simulink model "Traj2"  (R2025b)
settings: Solver=FixedStepAuto  StartTime=0.0  StopTime=inf  RelTol=1e-3
values from neighbouring files (symbols this model uses):
  K = [2.2361, 0, 0; 0, 2.8868, 2.5456]    [lq.m]
  vd_ref = v_refs    [lq.m]    (also in run_planner.m = zeros(N, 1))
  wd_ref = w_refs    [lq.m]    (also in run_planner.m = zeros(N, 1))
undefined symbols (not defined in the file or in its folder): L, P, theta0, theta_ref_unwrapped, Ts_ref, x0, y0
libraries: simulink x4, slpidlib x2
settings Model: Creator=mwali  LastModifiedBy=hassa
settings OptimizationCC: FunctionInliningControlUserFunctions=Never  FunctionInliningControlMWFunctions=Readability  FunctionInliningControlMWUserFunctions=Never  OptimizeBlockIOStorage=off  OptimizeDataStoreBuffers=off  BusAssignmentInplaceUpdate=off
settings DebuggingCC: SFUnexpectedBacktrackingDiag=warning  SFNoUnconditionalDefaultTransitionDiag=warning
settings RTWCC: GenerateReport=on  BuildConfiguration=Debug  LaunchReport=on
settings CodeAppCC: ForceParamTrailComments=on  MATLABSourceComments=on  EnableCustomComments=on
settings GRTTargetCC: MultiInstanceErrorCode=Warning  CombineSignalStateStructs=on  SupportVariableSizeSignals=on

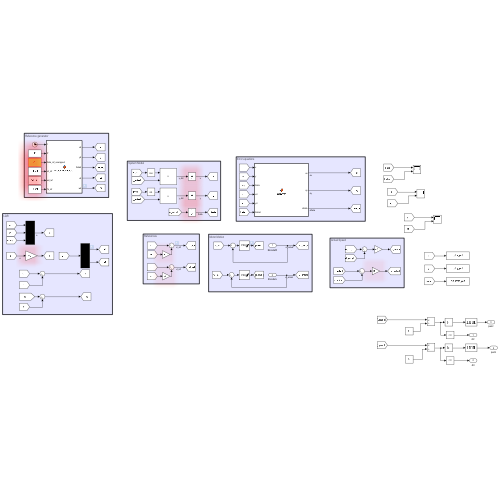
[thumbnail: Simulink's stored preview of the top-level diagram]
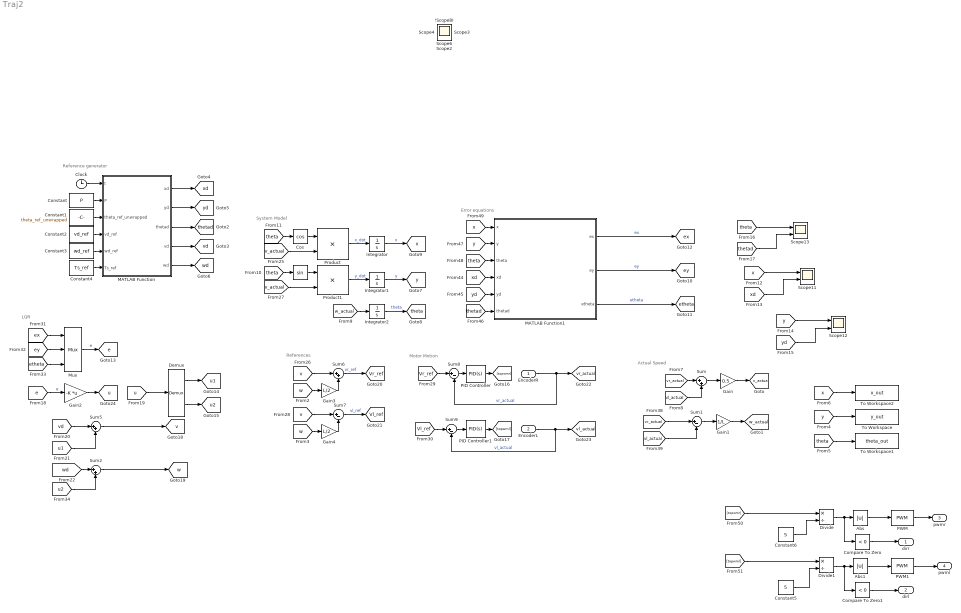
== system Traj2 ==
  note: Error equations
  note: Actual Speed
  note: Motor Motion
  note: References
  note: LQR
  note: System Model
  note: Reference generator
  EncoderR : Inport
  EncoderL : Inport  Port=2
  " " : Trigonometry
  Abs : Abs  SaturateOnIntegerOverflow=off
  Abs1 : Abs  SaturateOnIntegerOverflow=off
  Clock : Clock
  Compare To Zero : simulink/Logic and Bit Operations/Compare To Zero  relop=<  OutDataTypeStr=boolean
  Compare To Zero1 : simulink/Logic and Bit Operations/Compare To Zero  relop=<  OutDataTypeStr=boolean
  Constant : Constant  Value=P
  Constant1 : Constant  Value=theta_ref_unwrapped
  Constant2 : Constant  Value=vd_ref
  Constant3 : Constant  Value=wd_ref
  Constant4 : Constant  Value=Ts_ref
  Constant5 : Constant  Value=5
  Constant6 : Constant  Value=5
  Cos : Trigonometry  Operator=cos
  Demux : Demux  Outputs=2
  Divide : Product  Inputs=*/
  Divide1 : Product  Inputs=*/
  Gain : Gain  Gain=0.5
  Gain1 : Gain  Gain=1/L
  Gain2 : Gain  Gain=-K  Multiplication=Matrix(K*u)
  Gain3 : Gain  Gain=L/2
  Gain4 : Gain  Gain=L/2
  Integrator : Integrator  InitialCondition=x0
  Integrator1 : Integrator  InitialCondition=y0
  Integrator2 : Integrator  InitialCondition=theta0
  MATLAB Function : MATLAB Function  TreatAsAtomicUnit=on
  MATLAB Function1 : MATLAB Function  TreatAsAtomicUnit=on
  Mux : Mux  Inputs=3
  PID Controller : slpidlib/PID Controller  Controller=PID  Form=Parallel  TimeDomain=Continuous-time  UseExternalTs=off  SampleTime=-1  IntegratorMethod=Forward Euler  FilterMethod=Forward Euler  ControllerParametersSource=internal  P=5  I=20  UseKiTs=off  D=0  UseExternalDerivativeSource=off  N=100  UseFilter=on  TunerSelectOption=Transfer Function Based (PID Tuner App)  InitialConditionSource=internal  InitialConditionForIntegrator=0  InitialConditionForFilter=0  DifferentiatorICPrevScaledInput=0  ExternalReset=none  TrackingMode=off  Kt=1  LimitOutput=on  SatLimitsSource=internal  UpperSaturationLimit=5  LowerSaturationLimit=-5  LinearizeAsGain=on  AntiWindupMode=clamping  Kb=1  LimitIntegrator=off  UpperIntegratorSaturationLimit=inf  LowerIntegratorSaturationLimit=-inf  POutMin=[]  POutMax=[]  IOutMin=[]  IOutMax=[]  DOutMin=[]  DOutMax=[]  NOutMin=[]  NOutMax=[]  SumOutMin=[]  SumOutMax=[]  SaturationOutMin=[]  SaturationOutMax=[]  PParamMin=[]  PParamMax=[]  IParamMin=[]  IParamMax=[]  DParamMin=[]  DParamMax=[]  NParamMin=[]  NParamMax=[]  KbParamMin=[]  KbParamMax=[]  KtParamMin=[]  KtParamMax=[]  KbOutMin=[]  KbOutMax=[]  KtOutMin=[]  KtOutMax=[]  IntegratorOutMin=[]  IntegratorOutMax=[]  FilterOutMin=[]  FilterOutMax=[]  SumI1OutMin=[]  SumI1OutMax=[]  SumI2OutMin=[]  SumI2OutMax=[]  SumI3OutMin=[]  SumI3OutMax=[]  SumI4OutMin=[]  SumI4OutMax=[]  SumDOutMin=[]  SumDOutMax=[]  DifferentiatorOutMin=[]  DifferentiatorOutMax=[]  FilterDiffOutCoefMin=[]  FilterDiffOutCoefMax=[]  ReciprocalOutMin=[]  ReciprocalOutMax=[]  SumDenOutMin=[]  SumDenOutMax=[]  SumNumOutMin=[]  SumNumOutMax=[]  DivideOutMin=[]  DivideOutMax=[]  UdiffTsProdOutMin=[]  UdiffTsProdOutMax=[]  NTsProdOutMin=[]  NTsProdOutMax=[]  UintegralTsProdOutMin=[]  UintegralTsProdOutMax=[]  UngainTsProdOutMin=[]  UngainTsProdOutMax=[]  ClampingZeroOutDataTypeStr=Inherit: Inherit via back propagation  ClampingZeroOutMin=[]  ClampingZeroOutMax=[]  FilterDenConstantOutDataTypeStr=Inherit: Inherit via back propagation  FilterDenConstantOutMin=[]  FilterDenConstantOutMax=[]  PCopyOutDataTypeStr=Inherit: Inherit via back propagation  PCopyOutMin=[]  PCopyOutMax=[]  NCopyOutDataTypeStr=Inherit: Inherit via back propagation  NCopyOutMin=[]  NCopyOutMax=[]  IntegratorContinuousStateAttributes=''  IntegratorStateMustResolveToSignalObject=off  IntegratorRTWStateStorageClass=Auto  FilterContinuousStateAttributes=''  FilterStateMustResolveToSignalObject=off  FilterRTWStateStorageClass=Auto  ParallelPVariant=InternalParameters  IdealPVariant=Disabled  IVariant=InternalParameters  DVariant=InternalParameters  IntegratorVariant=Continuous  SatVariant=Enabled  AWVariant=ContClampingParallel  PCopyVariant=Disabled  TRVariant=Disabled  FdbkBlocksVariant=Forward  IdealPFdbkVariant=Disabled  SatFdbkVariant=Disabled  DerivativeFilterVariant=ContFilter  NVariant=InternalParameters  NCopyVariant=Disabled  FilterICVariant=InternalICsFilter  IntegratorICVariant=InternalICs  ExternalResetVariant=Disabled  TRSumVariant=Passthrough  SumFdbkVariant=Disabled  SumVariant=Sum_PID  TsampFilterVariant=InternalTs  TsampNgainVariant=Passthrough  TsampIntegralVariant=Disabled_SignalSpec  ExternalSaturationOutDataTypeStr=Inherit: Same as second input  DerivativeSourceVariant=ErrorSignal  PreIntVariant=InternalPreInt
  PID Controller1 : slpidlib/PID Controller  Controller=PID  Form=Parallel  TimeDomain=Continuous-time  UseExternalTs=off  SampleTime=-1  IntegratorMethod=Forward Euler  FilterMethod=Forward Euler  ControllerParametersSource=internal  P=5  I=20  UseKiTs=off  D=0  UseExternalDerivativeSource=off  N=100  UseFilter=on  TunerSelectOption=Transfer Function Based (PID Tuner App)  InitialConditionSource=internal  InitialConditionForIntegrator=0  InitialConditionForFilter=0  DifferentiatorICPrevScaledInput=0  ExternalReset=none  TrackingMode=off  Kt=1  LimitOutput=on  SatLimitsSource=internal  UpperSaturationLimit=5  LowerSaturationLimit=-5  LinearizeAsGain=on  AntiWindupMode=clamping  Kb=1  LimitIntegrator=off  UpperIntegratorSaturationLimit=inf  LowerIntegratorSaturationLimit=-inf  POutMin=[]  POutMax=[]  IOutMin=[]  IOutMax=[]  DOutMin=[]  DOutMax=[]  NOutMin=[]  NOutMax=[]  SumOutMin=[]  SumOutMax=[]  SaturationOutMin=[]  SaturationOutMax=[]  PParamMin=[]  PParamMax=[]  IParamMin=[]  IParamMax=[]  DParamMin=[]  DParamMax=[]  NParamMin=[]  NParamMax=[]  KbParamMin=[]  KbParamMax=[]  KtParamMin=[]  KtParamMax=[]  KbOutMin=[]  KbOutMax=[]  KtOutMin=[]  KtOutMax=[]  IntegratorOutMin=[]  IntegratorOutMax=[]  FilterOutMin=[]  FilterOutMax=[]  SumI1OutMin=[]  SumI1OutMax=[]  SumI2OutMin=[]  SumI2OutMax=[]  SumI3OutMin=[]  SumI3OutMax=[]  SumI4OutMin=[]  SumI4OutMax=[]  SumDOutMin=[]  SumDOutMax=[]  DifferentiatorOutMin=[]  DifferentiatorOutMax=[]  FilterDiffOutCoefMin=[]  FilterDiffOutCoefMax=[]  ReciprocalOutMin=[]  ReciprocalOutMax=[]  SumDenOutMin=[]  SumDenOutMax=[]  SumNumOutMin=[]  SumNumOutMax=[]  DivideOutMin=[]  DivideOutMax=[]  UdiffTsProdOutMin=[]  UdiffTsProdOutMax=[]  NTsProdOutMin=[]  NTsProdOutMax=[]  UintegralTsProdOutMin=[]  UintegralTsProdOutMax=[]  UngainTsProdOutMin=[]  UngainTsProdOutMax=[]  ClampingZeroOutDataTypeStr=Inherit: Inherit via back propagation  ClampingZeroOutMin=[]  ClampingZeroOutMax=[]  FilterDenConstantOutDataTypeStr=Inherit: Inherit via back propagation  FilterDenConstantOutMin=[]  FilterDenConstantOutMax=[]  PCopyOutDataTypeStr=Inherit: Inherit via back propagation  PCopyOutMin=[]  PCopyOutMax=[]  NCopyOutDataTypeStr=Inherit: Inherit via back propagation  NCopyOutMin=[]  NCopyOutMax=[]  IntegratorContinuousStateAttributes=''  IntegratorStateMustResolveToSignalObject=off  IntegratorRTWStateStorageClass=Auto  FilterContinuousStateAttributes=''  FilterStateMustResolveToSignalObject=off  FilterRTWStateStorageClass=Auto  ParallelPVariant=InternalParameters  IdealPVariant=Disabled  IVariant=InternalParameters  DVariant=InternalParameters  IntegratorVariant=Continuous  SatVariant=Enabled  AWVariant=ContClampingParallel  PCopyVariant=Disabled  TRVariant=Disabled  FdbkBlocksVariant=Forward  IdealPFdbkVariant=Disabled  SatFdbkVariant=Disabled  DerivativeFilterVariant=ContFilter  NVariant=InternalParameters  NCopyVariant=Disabled  FilterICVariant=InternalICsFilter  IntegratorICVariant=InternalICs  ExternalResetVariant=Disabled  TRSumVariant=Passthrough  SumFdbkVariant=Disabled  SumVariant=Sum_PID  TsampFilterVariant=InternalTs  TsampNgainVariant=Passthrough  TsampIntegralVariant=Disabled_SignalSpec  ExternalSaturationOutDataTypeStr=Inherit: Same as second input  DerivativeSourceVariant=ErrorSignal  PreIntVariant=InternalPreInt
  PWM : simulink/Discontinuities/PWM  DisableCoverage=on  Period=1/500  InitialDelay=0  DisallowZeroDutyCycle=off  RunAtFixedTimeIntervals=on  SampleTime=0.1
  PWM1 : simulink/Discontinuities/PWM  DisableCoverage=on  Period=1/500  InitialDelay=0  DisallowZeroDutyCycle=off  RunAtFixedTimeIntervals=on  SampleTime=0.1
  Product : Product
  Product1 : Product
  Scope11 : Scope  NumInputPorts=2
      settings: ActiveDisplayYMinimum=1.0833575360755143  ActiveDisplayYMaximum=10.249782175320373  DataLoggingVariableName=ScopeData11
  Scope12 : Scope  NumInputPorts=2
      settings: ActiveDisplayYMinimum=-0.0059982030677552256  ActiveDisplayYMaximum=10.053983827609798  DataLoggingVariableName=ScopeData12
  Scope13 : Scope  NumInputPorts=2
      settings: ActiveDisplayYMinimum=1.0311287515557852  ActiveDisplayYMaximum=3.7167864278411562  DataLoggingVariableName=ScopeData13
  Sum{,2,5..6} (4 alike) : Sum  Inputs=|++
  Sum{1,7..9} (4 alike) : Sum  Inputs=|+-
  To Workspace : ToWorkspace  VariableName=y_out  SampleTime=-1
  To Workspace1 : ToWorkspace  VariableName=theta_out  SampleTime=-1
  To Workspace2 : ToWorkspace  VariableName=x_out  SampleTime=-1
  dirr : Outport
  dirl : Outport  Port=2
  pwmr : Outport  Port=3
  pwml : Outport  Port=4
  Scope{,2..4,6,8,10} (7 alike) : Scope
      Scope settings: ActiveDisplayYMinimum=-0.11929  ActiveDisplayYMaximum=0.80552
      Scope10 settings: ActiveDisplayYMinimum=-1  ActiveDisplayYMaximum=1  DataLoggingVariableName=ScopeData10
      Scope2 settings: ActiveDisplayYMinimum=-1  ActiveDisplayYMaximum=1  DataLoggingVariableName=ScopeData2
      Scope3 settings: ActiveDisplayYMinimum=-1  ActiveDisplayYMaximum=1  DataLoggingVariableName=ScopeData3
      Scope4 settings: ActiveDisplayYMinimum=-1  ActiveDisplayYMaximum=1  DataLoggingVariableName=ScopeData4
      Scope6 settings: ActiveDisplayYMinimum=-1  ActiveDisplayYMaximum=1  DataLoggingVariableName=ScopeData6
      Scope8 settings: ActiveDisplayYMinimum=-5.1687  ActiveDisplayYMaximum=3.6193  DataLoggingVariableName=ScopeData8
  tag scope: Vl_ref=global, Vr_ref=global, e=global, etheta=global, ex=global, ey=global, theta=global, thetad=global, u1=global, u2=global, u=global, v=global, v_actual=global, vd=global, vl_actual=global, vr_actual=global, w=global, w_actual=global, wd=global, x=global, xd=global, y=global, yd=global
  wires:
  [y] -> To Workspace/1
  [theta] -> To Workspace1/1
  [x] -> To Workspace2/1
  Constant/1 -> MATLAB Function/2(P)
  Constant2/1 -> MATLAB Function/4(vd_ref)
  Clock/1 -> MATLAB Function/1(t)
  MATLAB Function/4(vd) -> [vd]
  Constant1/1 -> MATLAB Function/3(theta_ref_unwrapped)
  MATLAB Function/5(wd) -> [wd]
  MATLAB Function/3(thetad) -> [thetad]
  Constant4/1 -> MATLAB Function/6(Ts_ref)
  MATLAB Function/2(yd) -> [yd]
  MATLAB Function/1(xd) -> [xd]
  Constant3/1 -> MATLAB Function/5(wd_ref)
  [theta] -> " "/1
  " "/1 -> Product1/1
  Integrator/1 -> [x]  "x"
  Cos/1 -> Product/1
  Integrator2/1 -> [theta]  "theta"
  Product1/1 -> Integrator1/1  "y_dot"
  [w_actual] -> Integrator2/1
  Product/1 -> Integrator/1  "x_dot"
  [v_actual] -> Product/2
  [v_actual] -> Product1/2
  Integrator1/1 -> [y]  "y"
  [theta] -> Cos/1
  [e] -> Gain2/1  "e"
  [u1] -> Sum5/2
  Sum5/1 -> [v]
  [ey] -> Mux/2
  [ex] -> Mux/1
  [wd] -> Sum2/1
  Mux/1 -> [e]  "e"
  [etheta] -> Mux/3
  Demux/1 -> [u1]
  [u2] -> Sum2/2
  Gain2/1 -> [u]
  [vd] -> Sum5/1
  Demux/2 -> [u2]
  Sum2/1 -> [w]
  [u] -> Demux/1
  [v] -> Sum7/1
  [w] -> Gain4/1
  Sum6/1 -> [Vr_ref]  "vr_ref"
  Gain4/1 -> Sum7/2
  [w] -> Gain3/1
  [v] -> Sum6/1
  Sum7/1 -> [Vl_ref]  "vl_ref"
  Gain3/1 -> Sum6/2
  Sum8/1 -> PID Controller/1
  EncoderR/1 -> [vr_actual], Sum8/2  "vr_actual"
  [Vr_ref] -> Sum8/1
  [Vl_ref] -> Sum9/1
  PID Controller1/1 -> [topwml]
  Sum9/1 -> PID Controller1/1
  EncoderL/1 -> [vl_actual], Sum9/2  "vl_actual"
  PID Controller/1 -> [topwmr]
  Gain1/1 -> [w_actual]
  [vr_actual] -> Sum/1
  Gain/1 -> [v_actual]
  Sum/1 -> Gain/1
  [vr_actual] -> Sum1/1
  [vl_actual] -> Sum/2
  [vl_actual] -> Sum1/2
  Sum1/1 -> Gain1/1
  [x] -> Scope11/1
  [xd] -> Scope11/2
  [y] -> Scope12/1
  [yd] -> Scope12/2
  [theta] -> Scope13/1
  [thetad] -> Scope13/2
  [thetad] -> MATLAB Function1/6(thetad)
  MATLAB Function1/2(ey) -> [ey]  "ey"
  MATLAB Function1/3(etheta) -> [etheta]  "etheta"
  [x] -> MATLAB Function1/1(x)
  [yd] -> MATLAB Function1/5(yd)
  [xd] -> MATLAB Function1/4(xd)
  [y] -> MATLAB Function1/2(y)
  MATLAB Function1/1(ex) -> [ex]  "ex"
  [theta] -> MATLAB Function1/3(theta)
  [topwmr] -> Divide/1
  [topwml] -> Divide1/1
  Constant5/1 -> Divide1/2
  Constant6/1 -> Divide/2
  Divide/1 -> Abs/1, Compare To Zero/1
  Compare To Zero/1 -> dirr/1
  Abs/1 -> PWM/1
  Compare To Zero1/1 -> dirl/1
  Abs1/1 -> PWM1/1
  Divide1/1 -> Abs1/1, Compare To Zero1/1
  PWM/1 -> pwmr/1
  PWM1/1 -> pwml/1

== matlab function Traj2/MATLAB Function1 ==
  data: x input; ex output; y input; theta input; xd input; yd input; thetad input; ey output; etheta output
function [ex, ey, etheta] = calcError(x, y, theta, xd, yd, thetad)

dx = x - xd;
dy = y - yd;

ex =  cos(thetad)*dx + sin(thetad)*dy;
ey = -sin(thetad)*dx + cos(thetad)*dy;

etheta = atan2(sin(theta - thetad), cos(theta - thetad));

== matlab function Traj2/MATLAB Function ==
  data: t input; P input; theta_ref_unwrapped input; vd_ref input; wd_ref input; Ts_ref input; xd output; yd output; thetad output; vd output; wd output
function [xd, yd, thetad, vd, wd] = referenceGenerator(t, P, theta_ref_unwrapped, vd_ref, wd_ref, Ts_ref)

t_vec = (0:size(P,1)-1)' * Ts_ref;
t_clamped = min(max(t, t_vec(1)), t_vec(end));

xd     = interp1(t_vec, P(:,1), t_clamped, 'linear');
yd     = interp1(t_vec, P(:,2), t_clamped, 'linear');
thetad = interp1(t_vec, theta_ref_unwrapped, t_clamped, 'linear');
vd     = interp1(t_vec, vd_ref, t_clamped, 'linear');
wd     = interp1(t_vec, wd_ref, t_clamped, 'linear');

vd = max(vd, 0);
